simulink model "slave"  (R2022a)
settings: Solver=ode5  StartTime=0.0  StopTime=10  FixedStep=Ts  MaxStep=Ts  RelTol=1e-3
model workspace (MAT data in the model file):
  Sig = Simulink.Signal
  Sig.DataType = 'auto'
  Sig.Dimensions = -1
  Sig.DimensionsMode = 'auto'
  Sig.Complexity = 'auto'
  Sig.SampleTime = -1
  Sig.SamplingMode = 'auto'
  Sig1 = Simulink.Signal
  Sig1.DataType = 'auto'
  Sig1.Dimensions = -1
  Sig1.DimensionsMode = 'auto'
  Sig1.Complexity = 'auto'
  Sig1.SampleTime = -1
  Sig1.SamplingMode = 'auto'
  Sig2 = Simulink.Signal
  Sig2.DataType = 'auto'
  Sig2.Dimensions = -1
  Sig2.DimensionsMode = 'auto'
  Sig2.Complexity = 'auto'
  Sig2.SampleTime = -1
  Sig2.SamplingMode = 'auto'
  Sig3 = Simulink.Signal
  Sig3.DataType = 'auto'
  Sig3.Dimensions = -1
  Sig3.DimensionsMode = 'auto'
  Sig3.Complexity = 'auto'
  Sig3.SampleTime = -1
  Sig3.SamplingMode = 'auto'
  Sig4 = Simulink.Signal
  Sig4.DataType = 'auto'
  Sig4.Dimensions = -1
  Sig4.DimensionsMode = 'auto'
  Sig4.Complexity = 'auto'
  Sig4.SampleTime = -1
  Sig4.SamplingMode = 'auto'
  Ts = 0.001
  benv = Simulink.Parameter
  benv.Value = 13.5
  benv.DataType = 'auto'
  benv.Complexity = 'real'
  benv.Dimensions = [1 1]
  bm = Simulink.Parameter
  bm.Value = 0.1
  bm.DataType = 'auto'
  bm.Complexity = 'real'
  bm.Dimensions = [1 1]
  bms = Simulink.Parameter
  bms.Value = 23.5
  bms.DataType = 'auto'
  bms.Complexity = 'real'
  bms.Dimensions = [1 1]
  bs = Simulink.Parameter
  bs.Value = 0.1
  bs.DataType = 'auto'
  bs.Complexity = 'real'
  bs.Dimensions = [1 1]
  ctrl_slct = Simulink.Parameter
  ctrl_slct.Value = 1
  ctrl_slct.DataType = 'auto'
  ctrl_slct.Complexity = 'real'
  ctrl_slct.Dimensions = [1 1]
  fm = Simulink.Parameter
  fm.Value = 1
  fm.DataType = 'auto'
  fm.Complexity = 'real'
  fm.Dimensions = [1 1]
  kenv = Simulink.Parameter
  kenv.Value = 50
  kenv.DataType = 'auto'
  kenv.Complexity = 'real'
  kenv.Dimensions = [1 1]
  kms = Simulink.Parameter
  kms.Value = 150
  kms.DataType = 'auto'
  kms.Complexity = 'real'
  kms.Dimensions = [1 1]
  mm = Simulink.Parameter
  mm.Value = 1
  mm.DataType = 'auto'
  mm.Complexity = 'real'
  mm.Dimensions = [1 1]
  mms = Simulink.Parameter
  mms.Value = 0.5
  mms.DataType = 'auto'
  mms.Complexity = 'real'
  mms.Dimensions = [1 1]
  ms = Simulink.Parameter
  ms.Value = 1
  ms.DataType = 'auto'
  ms.Complexity = 'real'
  ms.Dimensions = [1 1]
  um = Simulink.Parameter
  um.Value = 0.1
  um.DataType = 'auto'
  um.Complexity = 'real'
  um.Dimensions = [1 1]
  us = Simulink.Parameter
  us.Value = 0.1
  us.DataType = 'auto'
  us.Complexity = 'real'
  us.Dimensions = [1 1]
  xbar = Simulink.Parameter
  xbar.Value = 0.1
  xbar.DataType = 'auto'
  xbar.Complexity = 'real'
  xbar.Dimensions = [1 1]
libraries: simulink x4
settings Model: PauseTimes=1.3  Creator=jueda3  LastModifiedBy=xzhao
settings SolverCC: AlgebraicLoopSolver=TrustRegion  AutoInsertRateTranBlk=on
settings DataIOCC: LimitDataPoints=on  SaveFormat=Array  SignalLoggingSaveFormat=ModelDataLogs  ReturnWorkspaceOutputs=off  SignalLoggingName=sigsOut
settings OptimizationCC: DefaultParameterBehavior=Inlined  EnhancedBackFolding=on  PassReuseOutputArgsAs=Individual arguments  ZeroExternalMemoryAtStartup=off  ZeroInternalMemoryAtStartup=off  OptimizeBlockOrder=speed  DifferentSizesBufferReuse=on  OptimizationCustomize=off  EfficientTunableParamExpr=on
settings DebuggingCC: SaveWithParameterizedLinksMsg=none  UnderspecifiedInitializationDetection=Classic  MergeDetectMultiDrivingBlocksExec=none  SignalResolutionControl=TryResolveAllWithWarning  MultiTaskDSMMsg=warning  MultiTaskCondExecSysMsg=none  ParameterTunabilityLossMsg=error  UnconnectedInputMsg=warning  UnconnectedOutputMsg=warning  UnconnectedLineMsg=warning  SFMachineParentedDataDiag=warning  ArithmeticOperatorsInVariantConditions=warning
settings HardwareCC: ProdBitPerPointer=32  ProdBitPerSizeT=32  ProdBitPerPtrDiffT=32  ProdLargestAtomicFloat=None  ProdIntDivRoundTo=Undefined  ProdEndianess=Unspecified  ProdWordSize=32  ProdHWDeviceType=32-bit Generic  TargetBitPerPointer=64  TargetBitPerSizeT=64  TargetBitPerPtrDiffT=64  TargetLongLongMode=on  TargetIntDivRoundTo=Zero  TargetEndianess=LittleEndian  TargetWordSize=64  TargetHWDeviceType=MATLAB Host  ProdEqTarget=off
settings ModelReferenceCC: PropagateSignalLabelsOutOfModel=off
settings SFSimCC: SimUseLocalCustomCode=off  MATLABDynamicMemAlloc=off  CustomCodeUndefinedFunction=UseInterfaceOnly
settings RTWCC: Description=Embedded Coder (host-based shared library target)  SystemTargetFile=ert_shrlib.tlc  TemplateMakefile=ert_default_tmf  RTWUseLocalCustomCode=off  DLArmComputeVersion=19.05
settings CodeAppCC: ForceParamTrailComments=on  IgnoreCustomStorageClasses=off  OperatorAnnotations=on  SimulinkDataObjDesc=on  SFDataObjDesc=on  InsertBlockDesc=on
settings STFCustomTargetCC: MultiwordLength=256  GenerateSampleERTMain=on  ParMdlRefBuildCompliant=on  CompOptLevelCompliant=on  CombineOutputUpdateFcns=on  ERTCustomFileBanners=on  SupportContinuousTime=off  SupportNonInlinedSFcns=off  RemoveResetFunc=on  MATLABClassNameForMDSCustomization=Simulink.SoftwareTarget.ERTCustomization  ModelStepFunctionPrototypeControlCompliant=on  GRTInterface=off  UseToolchainInfoCompliant=on  SystemTargetFile=ert_shrlib.tlc
settings ERTTargetCC: GenerateSampleERTMain=on  ConcurrentExecutionCompliant=off  CPPClassGenCompliant=off  InlinedParameterPlacement=NonHierarchical  ERTCustomFileTemplate=example_file_process.tlc
settings ConfigComp: CovMetricSettings=dw  CovSaveCumulativeToWorkspaceVar=on  CovSaveSingleToWorkspaceVar=on  CovExternalEMLEnable=off

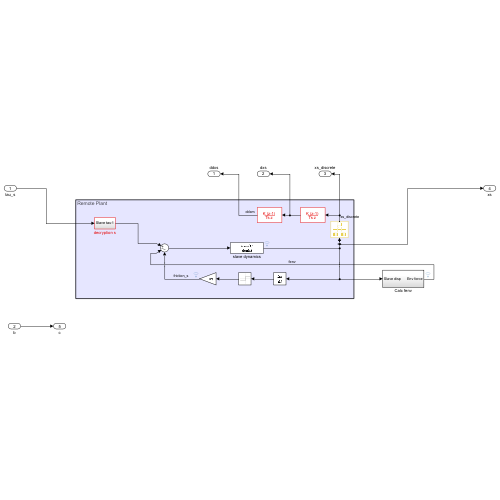
[thumbnail: Simulink's stored preview of the top-level diagram]
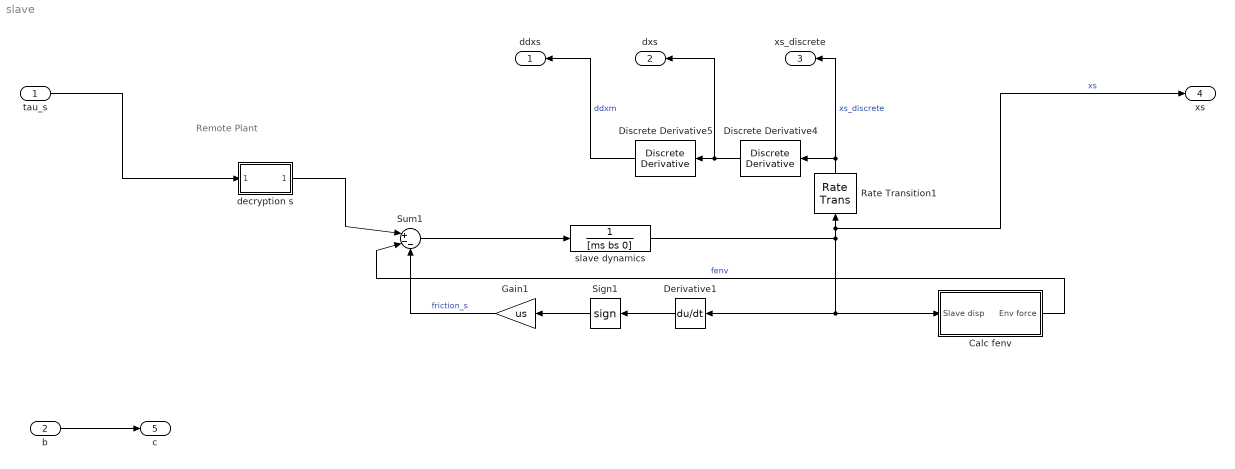
== system slave ==
  note: Remote Plant
  tau_s : Inport
  b : Inport  Port=2
  Calc fenv : Subsystem
  Derivative1 : Derivative  CoefficientInTFapproximation=0.01
  Discrete Derivative4 : simulink/Discrete/Discrete Derivative  gainval=1.0  ICPrevScaledInput=0.0  OutMin=[]  OutMax=[]  OutDataType=fixdt(1, 16)  OutScaling=2^-10  DoSatur=off
  Discrete Derivative5 : simulink/Discrete/Discrete Derivative  gainval=1.0  ICPrevScaledInput=0.0  OutMin=[]  OutMax=[]  OutDataType=fixdt(1, 16)  OutScaling=2^-10  DoSatur=off
  Gain1 : Gain  Gain=us
  Rate Transition1 : RateTransition  OutPortSampleTime=Ts
  Sign1 : Signum
  Sum1 : Sum  Inputs=|+--
  decryption s : Subsystem
  slave dynamics : TransferFcn  Denominator=[ms bs 0]
  ddxs : Outport
  dxs : Outport  Port=2
  xs_discrete : Outport  Port=3
  xs : Outport  Port=4
  c : Outport  Port=5
  wires:
  slave dynamics/1 -> xs/1, Rate Transition1/1, Calc fenv/1(Slave disp), Derivative1/1  "xs"
  Calc fenv/1(Env force) -> Sum1/2  "fenv"
  Sum1/1 -> slave dynamics/1
  Gain1/1 -> Sum1/3  "friction_s"
  Sign1/1 -> Gain1/1
  Rate Transition1/1 -> xs_discrete/1, Discrete Derivative4/1  "xs_discrete"
  decryption s/1(Out1) -> Sum1/1
  Discrete Derivative4/1 -> dxs/1, Discrete Derivative5/1
  Derivative1/1 -> Sign1/1
  Discrete Derivative5/1 -> ddxs/1  "ddxm"
  tau_s/1 -> decryption s/1(Slave tau)
  b/1 -> c/1

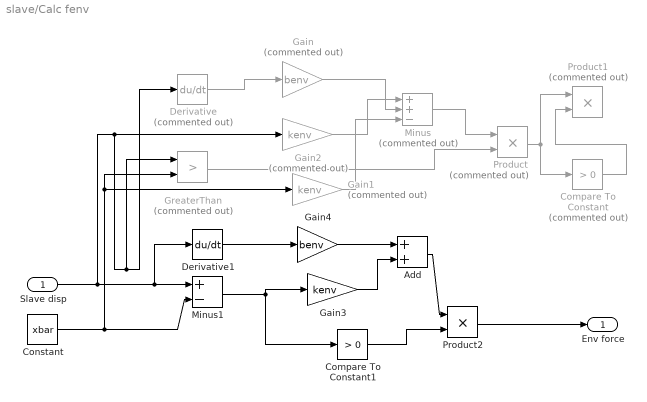
== system slave/Calc fenv ==
  Slave disp : Inport
  Add : Sum
  Compare To Constant : simulink/Logic and Bit Operations/Compare To Constant  Commented=on  relop=>  const=0  OutDataTypeStr=boolean
  Compare To Constant1 : simulink/Logic and Bit Operations/Compare To Constant  relop=>  const=0  OutDataTypeStr=boolean
  Constant : Constant  Value=xbar
  Derivative : Derivative  Commented=on
  Derivative1 : Derivative
  Gain : Gain  Commented=on  Gain=benv
  Gain1 : Gain  Commented=on  Gain=kenv
  Gain2 : Gain  Commented=on  Gain=kenv
  Gain3 : Gain  Gain=kenv
  Gain4 : Gain  Gain=benv
  GreaterThan : RelationalOperator  Commented=on  Operator=>  OutDataTypeStr=boolean  RndMeth=Simplest  InputSameDT=off
  Minus : Sum  Commented=on  Inputs=++-
  Minus1 : Sum  Inputs=+-
  Product : Product  Commented=on
  Product1 : Product  Commented=on
  Product2 : Product
  Env force : Outport
  wires:
  Slave disp/1 -> Gain2/1, Derivative/1, GreaterThan/1, Derivative1/1, Minus1/1
  Gain2/1 -> Minus/1
  Product/1 -> Compare To Constant/1, Product1/1
  Constant/1 -> GreaterThan/2, Gain1/1, Minus1/2
  GreaterThan/1 -> Product/2
  Gain1/1 -> Minus/3
  Minus/1 -> Product/1
  Derivative/1 -> Gain/1
  Gain/1 -> Minus/2
  Compare To Constant/1 -> Product1/2
  Minus1/1 -> Compare To Constant1/1, Gain3/1
  Gain3/1 -> Add/2
  Compare To Constant1/1 -> Product2/2
  Product2/1 -> Env force/1
  Derivative1/1 -> Gain4/1
  Gain4/1 -> Add/1
  Add/1 -> Product2/1

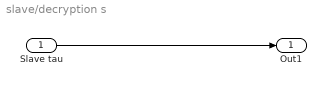
== system slave/decryption s ==
  Slave tau : Inport
  Out1 : Outport
  wires:
  Slave tau/1 -> Out1/1
